simulink model "Smart_EV_Charging_Station_Project_Simulation"  (R2024b)
settings: Solver=ode23tb  StartTime=0.0  StopTime=4  RelTol=1e-12
undefined symbols (not defined in the file): Ion, Lithium
libraries: spsSeriesRLCBranchLib x34, spsPWMGeneratorDCDCLib x12, spsIdealSwitchLib x12, slpidlib x11, spsGroundLib x10, spsMosfetLib x10, spsIGBTDiodeLib x8, spsDiodeLib x7, spsVoltageMeasurementLib x7, spsBatteryLib x6, spsIGBTLib x6, spsThyristorLib x6
(part 1 of 3)
settings Model: Creator=HP  LastModifiedBy=mahad
settings SolverCC: AlgebraicLoopSolver=TrustRegion
settings DataIOCC: ReturnWorkspaceOutputs=off
settings DebuggingCC: UnconnectedInputMsg=warning  UnconnectedOutputMsg=warning  UnconnectedLineMsg=warning  ArithmeticOperatorsInVariantConditions=warning
settings ModelReferenceCC: EnableRefExpFcnMdlSchedulingChecks=on
settings SFSimCC: SimUseLocalCustomCode=off  CustomCodeUndefinedFunction=UseInterfaceOnly
settings RTWCC: RTWUseLocalCustomCode=off  GPUComputeCapability=3.5
settings CodeAppCC: StateflowObjectComments=on
settings SimscapeCC: SimscapeNormalizeSystem=off

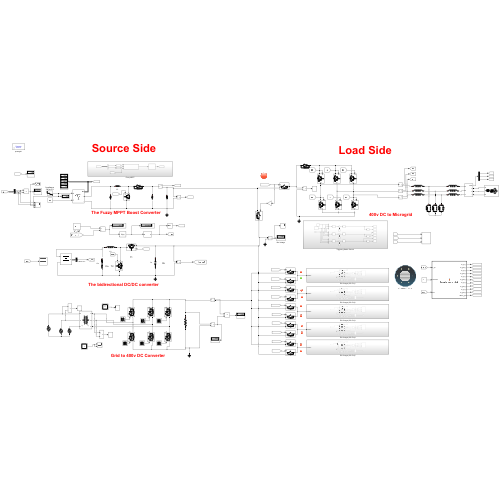
[thumbnail: Simulink's stored preview of the top-level diagram]
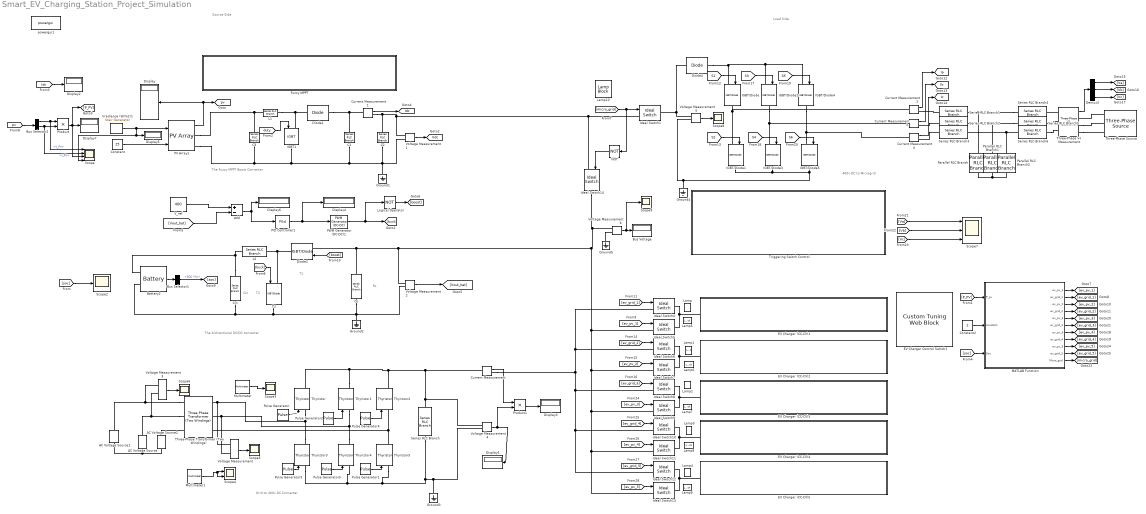
== system Smart_EV_Charging_Station_Project_Simulation ==
  note: The bidirectional DC/DC converter
  note: The Fuzzy MPPT Boost Converter
  note: Grid to 400v DC Converter
  note: 400v DC to Microgrid
  note: Source Side
  note: Load Side
  note: T1
  note: T2
  note: Cin
  note: RL
  AC Voltage Source : spsACVoltageSourceLib/AC Voltage Source  Amplitude=120*1.414  Phase=-120  Frequency=60  SampleTime=0  Measurements=Voltage  BusType=swing  Pref=10e3  Qref=0  Qmin=-inf  Qmax=+inf
  AC Voltage Source1 : spsACVoltageSourceLib/AC Voltage Source  Amplitude=120*1.414  Phase=0  Frequency=60  SampleTime=0  Measurements=Voltage  BusType=swing  Pref=10e3  Qref=0  Qmin=-inf  Qmax=+inf
  AC Voltage Source2 : spsACVoltageSourceLib/AC Voltage Source  Amplitude=120*1.414  Phase=-240  Frequency=60  SampleTime=0  Measurements=Voltage  BusType=swing  Pref=10e3  Qref=0  Qmin=-inf  Qmax=+inf
  Add : Sum  Inputs=+-
  Battery2 : spsBatteryLib/Battery  BatType=Lithium-Ion  NomV=400  NomQ=1400  SOC=50  Batt_Tr=0.01  PresetModel=on  MaxQ=1400  MinV=300  FullV=465.5949  Dis_rate=608.6957  R=0.0028571  Normal_OP=1266.087  expZone="[432.1543      68.78261]"
      settings: LibrarySourceBlock=electricdrivelib/Extra Sources/Battery
  Bus Selector1 : BusSelector  OutputSignals=SOC (%)
  Bus Selector2 : BusSelector  OutputSignals=V_PV,I_PV
  Bus Voltage : Display
  C1 : spsSeriesRLCBranchLib/Series RLC Branch  LConnTagsString=__new0  RConnTagsString=__new0  BranchType=C  Resistance=1.0  Inductance=1.0  SetiL0=off  InitialCurrent=0  Capacitance=0.04  Setx0=off  InitialVoltage=0  Measurements=None
  C2 : spsSeriesRLCBranchLib/Series RLC Branch  LConnTagsString=__new0  RConnTagsString=__new0  BranchType=R  Resistance=0.28  Inductance=1.0  SetiL0=off  InitialCurrent=0  Capacitance=100e-6  Setx0=off  InitialVoltage=0  Measurements=Branch voltage
  C3 : spsSeriesRLCBranchLib/Series RLC Branch  LConnTagsString=__new0  RConnTagsString=__new0  BranchType=C  Resistance=1.0  Inductance=1.0  SetiL0=off  InitialCurrent=0  Capacitance=0.00018  Setx0=off  InitialVoltage=0  Measurements=None
  Cin : spsSeriesRLCBranchLib/Series RLC Branch  LConnTagsString=__new0  RConnTagsString=__new0  BranchType=RC  Resistance=0.0000005  Inductance=3e-3  SetiL0=off  InitialCurrent=0  Capacitance=0.015  Setx0=off  InitialVoltage=0  Measurements=None
  Co : spsSeriesRLCBranchLib/Series RLC Branch  LConnTagsString=__new0  RConnTagsString=__new0  BranchType=C  Resistance=1  Inductance=3e-3  SetiL0=off  InitialCurrent=0  Capacitance=0.01  Setx0=off  InitialVoltage=0  Measurements=None
  Constant : Constant  Value=25
  Constant2 : Constant
  Current Measurement{,1..4} (5 alike) : spsCurrentMeasurementLib/Current Measurement  PhasorSimulation=off  OutputType=Complex  PSBequivalent=0
  Demux3 : Demux  Outputs=3
  Diode1 : spsDiodeLib/Diode  Ron=0.001  Lon=0  Vf=0.8  IC=0  UseSnubber=0  Rs=500  Cs=250e-9  Measurements=off
  Diode2 : spsIGBTDiodeLib/IGBT//Diode  Ron=1e-3  Rs=1e5  Cs=inf  Measurements=off
  Diode4 : spsDiodeLib/Diode  Ron=0.001  Lon=0  Vf=0.8  IC=0  UseSnubber=0  Rs=500  Cs=250e-9  Measurements=off
  Display{,1..7} (8 alike) : Display
  EV Charger (CC-CV)1 : Subsystem
  EV Charger (CC-CV)2 : Subsystem
  EV Charger (CC-CV)3 : Subsystem
  EV Charger (CC-CV)4 : Subsystem
  EV Charger (CC-CV)5 : Subsystem
  EV Charger Control Switch1 : CustomTuningWebBlock  LabelPosition=Bottom  ShowInitialText=on  Configuration="{\"components\":[{\"name\":\"RotarySwitchComponent\",\"settings\":{\"arcAngle\":300,\"arcAngleOffset\":120,\"handle\":{\"size\":[150,150],\"src\":\"data:image\\/svg+xml;base64,PHN2ZyBpZD0iTGF5ZXJfMSIgZGF0YS1uYW1lPSJMYXllciAxIiB4bWxucz0iaHR0cDovL3d3dy53My5vcmcvMjAwMC9zdmciIHhtbG5zOnhsaW5rPSJodHRwOi8vd3d3LnczLm9yZy8xOTk5L3hsaW5rIiB2aWV3Qm94PSIwIDAgMTIxIDEyMSI+PGRlZnM+PHN0eWxlPi5jbHMtMXtmaWxsOnVybCgjbGluZWFyLWdyYWRpZW50KTt9LmNscy0yLC5jbHMtM3tmaWxsOiNkMWQxZDE7fS5jbHMtM3tzdHJva2U6I2I3YjdiNztzdHJva2UtbWl0ZXJsaW1pdDoxMDtzdHJva2Utd2lkdGg6MC4yNXB4O30uY2xzLTR7ZmlsbDojZjMwMDAwO30uY2xzLTV7ZmlsbDojZjIxNzY3O308L3N0eWxlPjxsaW5lYXJHcmFkaWVudCBpZD0ibGluZWFyLWdyYWRpZW50IiB4MT0iNjAuNSIgeTE9IjEyMC41IiB4Mj0iNjAuNSIgeTI9IjAuNSIgZ3JhZGllbnRVbml0cz0idXNlclNwYWNlT25Vc2UiPjxzdG9wIG9mZnNldD0iMCIgc3RvcC1jb2xvcj0iI2QxZDFkMSIvPjxzdG9wIG9mZnNldD0iMC4xIiBzdG9wLWNvbG9yPSIjY2VjZWNlIi8+PHN0b3Agb2Zmc2V0PSIwLjE5IiBzdG9wLWNvbG9yPSIjYzNjM2MzIi8+PHN0b3Agb2Zmc2V0PSIwLjI4IiBzdG9wLWNvbG9yPSIjYjFiMWIxIi8+PHN0b3Agb2Zmc2V0PSIwLjM2IiBzdG9wLWNvbG9yPSIjOTg5ODk4Ii8+PHN0b3Agb2Zmc2V0PSIwLjQ0IiBzdG9wLWNvbG9yPSIjNzg3ODc4Ii8+PHN0b3Agb2Zmc2V0PSIwLjQ2IiBzdG9wLWNvbG9yPSIjNmI2YjZiIi8+PHN0b3Agb2Zmc2V0PSIwLjU0IiBzdG9wLWNvbG9yPSIjNmI2YjZiIi8+PHN0b3Agb2Zmc2V0PSIwLjU2IiBzdG9wLWNvbG9yPSIjNzY3Njc2Ii8+PHN0b3Agb2Zmc2V0PSIwLjY0IiBzdG9wLWNvbG9yPSIjOTc5Nzk3Ii8+PHN0b3Agb2Zmc2V0PSIwLjcyIiBzdG9wLWNvbG9yPSIjYjBiMGIwIi8+PHN0b3Agb2Zmc2V0PSIwLjgxIiBzdG9wLWNvbG9yPSIjYzNjM2MzIi8+PHN0b3Agb2Zmc2V0PSIwLjkiIHN0b3AtY29sb3I9IiNjZGNkY2QiLz48c3RvcCBvZmZzZXQ9IjEiIHN0b3AtY29sb3I9IiNkMWQxZDEiLz48L2xpbmVhckdyYWRpZW50PjwvZGVmcz48Y2lyY2xlIGNsYXNzPSJjbHMtMSIgY3g9IjYwLjUiIGN5PSI2MC41IiByPSI2MCIvPjxwYXRoIGNsYXNzPSJjbHMtMiIgZD0iTTYwLjUsMUE1OS41LDU5LjUsMCwxLDEsMSw2MC41LDU5LjU3LDU5LjU3LDAsMCwxLDYwLjUsMW0wLTFBNjAuNSw2MC41LDAsMSwwLDEyMSw2MC41LDYwLjUsNjAuNSwwLDAsMCw2MC41LDBaIi8+PHJlY3QgY2xhc3M9ImNscy0zIiB4PSIwLjUiIHk9IjUxLjUiIHdpZHRoPSIxMjAiIGhlaWdodD0iMTgiIHJ4PSIzLjA0Ii8+PHJlY3QgY2xhc3M9ImNscy00IiB4PSI1Ljc1IiB5PSI1OC43NSIgd2lkdGg9IjE2IiBoZWlnaHQ9IjMiLz48cGF0aCBjbGFzcz0iY2xzLTUiIGQ9Ik0yMS4yNSw1OS4yNXYyaC0xNXYtMmgxNW0xLTFoLTE3djRoMTd2LTRaIi8+PC9zdmc+\"},\"handleOffset\":[0,0],\"handleOrientation\":180,\"handlePosition\":[0,0,1,1],\"handleSize\":{\"height\":0.5,\"width\":0.5},\"labelRadius\":0.36,\"position\":[0,0,1,1],\"states\":[{\"Label\":{\"color\":[0,0,0,1],\"icon\":{\"size\":[0,0],\"src\":[],\"srcOrientation\":\"Right\"},\"iconOffset\":0,\"iconPlacement\":\"left\",\"opacity\":1,\"position\":[0.7345552884615385,0.6796274038461538],\"show\":true,\"text\":{\"content\":\"0\",\"font\":\"Helvetica\"}},\"Value\":0},{\"Label\":{\"color\":[0,0,0,1],\"icon\":{\"size\":[0,0],\"src\":[],\"srcOrientation\":\"Right\"},\"iconOffset\":0,\"iconPlacement\":\"left\",\"opacity\":1,\"position\":[0.35757211538461536,0.7603966346153846],\"show\":true,\"text\":{\"content\":\"1\",\"font\":\"Helvetica\"}},\"Value\":1},{\"Label\":{\"color\":[0,0,0,1],\"icon\":{\"size\":[0,0],\"src\":[],\"srcOrientation\":\"Right\"},\"iconOffset\":0,\"iconPlacement\":\"left\",\"opacity\":1,\"position\":[0.09603365384615385,0.46033653846153844],\"show\":true,\"text\":{\"content\":\"2\",\"font\":\"Helvetica\"}},\"Value\":2},{\"Label\":{\"color\":[0,0,0,1],\"icon\":{\"size\":[0,0],\"src\":[],\"srcOrientation\":\"Right\"},\"iconOffset\":0,\"iconPlacement\":\"left\",\"opacity\":1,\"position\":[0.36532451923076925,0.1180889423076923],\"show\":true,\"text\":{\"content\":\"3\",\"font\":\"Helvetica\"}},\"Value\":3},{\"Label\":{\"color\":[0,0,0,1],\"icon\":{\"size\":[0,0],\"src\":[],\"srcOrientation\":\"Right\"},\"iconOffset\":0,\"iconPlacement\":\"left\",\"opacity\":1,\"position\":[0.7191706730769231,0.19501201923076922],\"show\":true,\"text\":{\"content\":\"4\",\"font\":\"Helvetica\"}},\"Value\":4},{\"Label\":{\"color\":[0,0,0,1],\"icon\":{\"size\":[0,0],\"src\":[],\"srcOrientation\":\"Right\"},\"iconOffset\":0,\"iconPlacement\":\"left\",\"opacity\":1,\"position\":[0.7191706730769231,0.19501201923076922],\"show\":true,\"text\":{\"content\":\"5\",\"font\":\"Helvetica\"}},\"Value\":5}],\"tickRadius\":0.32}},{\"name\":\"BackgroundImageComponent\",\"settings\":{\"image\":{\"size\":[155,150],\"src\":\"data:image\\/svg+xml;base64,PD94bWwgdmVyc2lvbj0iMS4wIiBlbmNvZGluZz0idXRmLTgiPz4NCjwhLS0gR2VuZXJhdG9yOiBBZG9iZSBJbGx1c3RyYXRvciAyNS4wLjAsIFNWRyBFeHBvcnQgUGx1Zy1JbiAuIFNWRyBWZXJzaW9uOiA2LjAwIEJ1aWxkIDApICAtLT4NCjxzdmcgdmVyc2lvbj0iMS4xIg0KCSBpZD0iTGF5ZXJfMl8xXyIgeG1sbnM6Y2M9Imh0dHA6Ly9jcmVhdGl2ZWNvbW1vbnMub3JnL25zIyIgeG1sbnM6ZGM9Imh0dHA6Ly9wdXJsLm9yZy9kYy9lbGVtZW50cy8xLjEvIiB4bWxuczppbmtzY2FwZT0iaHR0cDovL3d3dy5pbmtzY2FwZS5vcmcv ...(+4184 chars)\",\"srcOrientation\":\"Right\"},\"position\":[0,0,1,1],\"scaleMode\":\"0\"}},{\"name\":\"ForegroundImageComponent\",\"settings\":{\"image\":{\"size\":[0,0],\"src\":\"default\",\"srcOrientation\":[]},\"isForeground\":1,\"position\":[0,0,1,1],\"scaleMode\":\"0\"}}],\"settings\":{\"BindingType\":\"param\",\"backgroundColor\":[0,0,255,\"1\"],\"backgroundOffset\":1,\"fixedAspectRatio\":\"on\",\"image\":{\"size\":[150,150],\"src\":\"data:image\\/svg+xml;base64,PD94bWwgdmVyc2lvbj0iMS4wIiBlbmNvZGluZz0iVVRGLTgiIHN0YW5kYWxvbmU9Im5vIj8+CjwhLS0gR2VuZXJhdG9yOiBBZG9iZSBJbGx1c3RyYXRvciAxOS4yLjEsIFNWRyBFeHBvcnQgUGx1Zy1JbiAuIFNWRyBWZXJzaW9uOiA2LjAwIEJ1aWxkIDApICAtLT4KCjxzdmcKICAgeG1sbnM6ZGM9Imh0dHA6Ly9wdXJsLm9yZy9kYy9lbGVtZW50cy8xLjEvIgogICB4bWxuczpjYz0iaHR0cDovL2NyZWF0aXZlY29tbW9ucy5vcmcvbnMjIgogICB4bWxuczpyZGY9Imh0dHA6Ly93d3cudzMub3JnLzE5OTkvMDIvMjItcmRmLXN5bnRh ...(+9660 chars)\"},\"showBackgroundColor\":false,\"variant\":\"rotarySwitch\",\"version\":\"R2023a\"},\"type\":\"RotarySwitch\"}"
  Fuzzy MPPT : Subsystem
  Ground{1..5} (5 alike) : spsGroundLib/Ground  LConnTagsString=a
  IGBT/Diode{,1..5} (6 alike) : spsIGBTDiodeLib/IGBT//Diode  Ron=1e-3  Rs=1e5  Cs=inf  Measurements=off
  IGBT1 : spsIGBTLib/IGBT  Ron=0.001  Lon=0  Vf=0  Tf=0  Tt=0  IC=0  Rs=1e5  Cs=inf  Measurements=off
  Ideal Switch{1,4..14} (12 alike) : spsIdealSwitchLib/Ideal Switch  Ron=0.001  Lon=0  IC=0  Rs=1e5  Cs=inf  Measurements=off
  Irradiance (W/m2)1 : spsStairGeneratorLib/Stair Generator  t=[0, 1, 2,3]  e=[1,0.8, 0.7, 0.6]*1000  Ts=0.0001
  L1 : spsSeriesRLCBranchLib/Series RLC Branch  LConnTagsString=__new0  RConnTagsString=__new0  BranchType=L  Resistance=0.005  Inductance=1.8e-05  SetiL0=off  InitialCurrent=0  Capacitance=1e-6  Setx0=off  InitialVoltage=0  Measurements=None
  L2 : spsSeriesRLCBranchLib/Series RLC Branch  LConnTagsString=__new0  RConnTagsString=__new0  BranchType=L  Resistance=.25  Inductance=4e-4  SetiL0=off  InitialCurrent=0  Capacitance=1e-6  Setx0=off  InitialVoltage=0  Measurements=None
  Lamp{,1..10} (11 alike) : LampBlock  LabelPosition=Hide
  Logical Operator : Logic  Operator=NOT  AllPortsSameDT=off  OutDataTypeStr=boolean
  MATLAB Function : MATLAB Function  TreatAsAtomicUnit=on
  Multimeter : spsMultimeterLib/Multimeter  L=11  sel=[2 3]  yselected={}  Gain=[1 1]  OutputType=Complex  PlotAtSimulationStop=off  PhasorSimulation=off
  Multimeter1 : spsMultimeterLib/Multimeter  L=11  sel=4  yselected={}  Gain=1  OutputType=Complex  PlotAtSimulationStop=off  PhasorSimulation=off
  NOT : Logic  Operator=NOT  IconShape=distinctive  AllPortsSameDT=off  OutDataTypeStr=boolean
  PID Controller1 : slpidlib/PID Controller  Controller=PI  Form=Parallel  TimeDomain=Continuous-time  UseExternalTs=off  SampleTime=-1  IntegratorMethod=Forward Euler  FilterMethod=Forward Euler  ControllerParametersSource=internal  P=0.00001  I=0.005  UseKiTs=off  D=0  UseExternalDerivativeSource=off  N=100  UseFilter=on  TunerSelectOption=Transfer Function Based (PID Tuner App)  InitialConditionSource=internal  InitialConditionForIntegrator=0  InitialConditionForFilter=0  DifferentiatorICPrevScaledInput=0  ExternalReset=none  TrackingMode=off  Kt=1  LimitOutput=off  SatLimitsSource=internal  UpperSaturationLimit=inf  LowerSaturationLimit=-inf  LinearizeAsGain=on  AntiWindupMode=none  Kb=1  LimitIntegrator=off  UpperIntegratorSaturationLimit=inf  LowerIntegratorSaturationLimit=-inf  POutMin=[]  POutMax=[]  IOutMin=[]  IOutMax=[]  DOutMin=[]  DOutMax=[]  NOutMin=[]  NOutMax=[]  SumOutMin=[]  SumOutMax=[]  SaturationOutMin=[]  SaturationOutMax=[]  PParamMin=[]  PParamMax=[]  IParamMin=[]  IParamMax=[]  DParamMin=[]  DParamMax=[]  NParamMin=[]  NParamMax=[]  KbParamMin=[]  KbParamMax=[]  KtParamMin=[]  KtParamMax=[]  KbOutMin=[]  KbOutMax=[]  KtOutMin=[]  KtOutMax=[]  IntegratorOutMin=[]  IntegratorOutMax=[]  FilterOutMin=[]  FilterOutMax=[]  SumI1OutMin=[]  SumI1OutMax=[]  SumI2OutMin=[]  SumI2OutMax=[]  SumI3OutMin=[]  SumI3OutMax=[]  SumI4OutMin=[]  SumI4OutMax=[]  SumDOutMin=[]  SumDOutMax=[]  DifferentiatorOutMin=[]  DifferentiatorOutMax=[]  FilterDiffOutCoefMin=[]  FilterDiffOutCoefMax=[]  ReciprocalOutMin=[]  ReciprocalOutMax=[]  SumDenOutMin=[]  SumDenOutMax=[]  SumNumOutMin=[]  SumNumOutMax=[]  DivideOutMin=[]  DivideOutMax=[]  UdiffTsProdOutMin=[]  UdiffTsProdOutMax=[]  NTsProdOutMin=[]  NTsProdOutMax=[]  UintegralTsProdOutMin=[]  UintegralTsProdOutMax=[]  UngainTsProdOutMin=[]  UngainTsProdOutMax=[]  ClampingZeroOutDataTypeStr=Inherit: Inherit via back propagation  ClampingZeroOutMin=[]  ClampingZeroOutMax=[]  FilterDenConstantOutDataTypeStr=Inherit: Inherit via back propagation  FilterDenConstantOutMin=[]  FilterDenConstantOutMax=[]  PCopyOutDataTypeStr=Inherit: Inherit via back propagation  PCopyOutMin=[]  PCopyOutMax=[]  NCopyOutDataTypeStr=Inherit: Inherit via back propagation  NCopyOutMin=[]  NCopyOutMax=[]  IntegratorContinuousStateAttributes=''  IntegratorStateMustResolveToSignalObject=off  IntegratorRTWStateStorageClass=Auto  FilterContinuousStateAttributes=''  FilterStateMustResolveToSignalObject=off  FilterRTWStateStorageClass=Auto  ParallelPVariant=InternalParameters  IdealPVariant=Disabled  IVariant=InternalParameters  DVariant=Disabled  IntegratorVariant=Continuous  SatVariant=Disabled  AWVariant=Passthrough  PCopyVariant=Disabled  TRVariant=Disabled  FdbkBlocksVariant=Forward  IdealPFdbkVariant=Disabled  SatFdbkVariant=Disabled  DerivativeFilterVariant=Disabled  NVariant=Disabled  NCopyVariant=Disabled_SignalSpec  FilterICVariant=Disabled  IntegratorICVariant=InternalICs  ExternalResetVariant=Disabled  TRSumVariant=Passthrough  SumFdbkVariant=Disabled  SumVariant=Sum_PI  TsampFilterVariant=InternalTs  TsampNgainVariant=Passthrough  TsampIntegralVariant=Disabled_SignalSpec  ExternalSaturationOutDataTypeStr=Inherit: Same as second input  DerivativeSourceVariant=Disabled  PreIntVariant=InternalPreInt
  PV Array1 : spsPVArrayLib/PV Array  Npar=200  Nser=8  PlotType=array @ 25 deg.C & specified irradiances  S_vec="[ 1000  800  600 400 200 ]"  Temp_C_vec="[ 45 25  ]"  ModuleName=Canadian Solar Inc. CS3U-375MS-AG  PlotWhenSelected=off  Pm=375.314  Ncell=72  Voc=47.6  Isc=9.93  Vm=39.8  Im=9.43  beta_Voc_pc=-0.293  alpha_Isc_pc=0.035005  beta_Voc=-0.13947  alpha_Isc=0.003476  IL=9.9881  I0=2.473e-11  nI=0.96345  Rsh=294.0017  Rs=0.24088  RobustModel=off  RobustCellTemperature=313.3991  BAL=off  Tc=1e-6  Tfilter=1e-5
  PWM Generator (DC-DC)1 : spsPWMGeneratorDCDCLib/PWM Generator (DC-DC)  Fsw=10000  Ts=0
  Parallel RLC Branch : spsParallelRLCBranchLib/Parallel RLC Branch  LConnTagsString=a  RConnTagsString=__new0  BranchType=RC  Resistance=5.34  Inductance=1e-3  SetiL0=off  InitialCurrent=0  Capacitance=9.94e-6  Setx0=off  InitialVoltage=0  Measurements=None
  Parallel RLC Branch1 : spsParallelRLCBranchLib/Parallel RLC Branch  LConnTagsString=a  RConnTagsString=__new0  BranchType=RC  Resistance=5.34  Inductance=1e-3  SetiL0=off  InitialCurrent=0  Capacitance=9.94e-6  Setx0=off  InitialVoltage=0  Measurements=None
  Parallel RLC Branch2 : spsParallelRLCBranchLib/Parallel RLC Branch  LConnTagsString=a  RConnTagsString=__new0  BranchType=RC  Resistance=5.34  Inductance=1e-3  SetiL0=off  InitialCurrent=0  Capacitance=9.94e-6  Setx0=off  InitialVoltage=0  Measurements=None
  Product : Product
  Product1 : Product
  Pulse Generator : DiscretePulseGenerator  PulseType=Time based  Period=0.016  PulseWidth=33.33  PhaseDelay=60*0.016/360
  Pulse Generator1 : DiscretePulseGenerator  PulseType=Time based  Period=0.016  PulseWidth=33.33  PhaseDelay=120*0.016/360
  Pulse Generator2 : DiscretePulseGenerator  PulseType=Time based  Period=0.016  PulseWidth=33.33  PhaseDelay=180*0.016/360
  Pulse Generator3 : DiscretePulseGenerator  PulseType=Time based  Period=0.016  PulseWidth=33.33  PhaseDelay=240*0.016/360
  Pulse Generator4 : DiscretePulseGenerator  PulseType=Time based  Period=0.016  PulseWidth=33.33  PhaseDelay=300*0.016/360
  Pulse Generator5 : DiscretePulseGenerator  PulseType=Time based  Period=0.016  PulseWidth=33.33  PhaseDelay=360*0.016/360
  Scope : Scope  NumInputPorts=4
  Scope{2..3,5..6,8..9} (6 alike) : Scope
  Scope4 : Scope  NumInputPorts=2
  Scope7 : Scope  NumInputPorts=3
  Series RLC Branch : spsSeriesRLCBranchLib/Series RLC Branch  LConnTagsString=__new0  RConnTagsString=__new0  BranchType=R  Resistance=10  Inductance=1e-3  SetiL0=off  InitialCurrent=0  Capacitance=1e-6  Setx0=off  InitialVoltage=0  Measurements=Branch voltage and current
  Series RLC Branch{1,4..6} (4 alike) : spsSeriesRLCBranchLib/Series RLC Branch  LConnTagsString=__new0  RConnTagsString=__new0  BranchType=L  Resistance=1e-3  Inductance=5.1e-3  SetiL0=off  InitialCurrent=0  Capacitance=1e-6  Setx0=off  InitialVoltage=0  Measurements=None
  Series RLC Branch2 : spsSeriesRLCBranchLib/Series RLC Branch  LConnTagsString=__new0  RConnTagsString=__new0  BranchType=L  Resistance=1e-3  Inductance=5.1e-6  SetiL0=off  InitialCurrent=0  Capacitance=1e-6  Setx0=off  InitialVoltage=0  Measurements=None
  Series RLC Branch3 : spsSeriesRLCBranchLib/Series RLC Branch  LConnTagsString=__new0  RConnTagsString=__new0  BranchType=L  Resistance=1e-3  Inductance=5.1e-6  SetiL0=off  InitialCurrent=0  Capacitance=1e-6  Setx0=off  InitialVoltage=0  Measurements=None
  T2 : spsIGBTDiodeLib/IGBT//Diode  Ron=1e-3  Rs=1e5  Cs=inf  Measurements=off
  Three-Phase Transformer (Two Windings) : spsThreePhaseTransformerTwoWindingsLib/Three-Phase Transformer (Two Windings)  Winding1Connection=Yg  Winding2Connection=Yg  CoreType=Three single-phase transformers  SetSaturation=off  Hysteresis=off  DataFile='hysteresis'  SetInitialFlux=off  Measurements=None  UNITS=pu  NominalPower=[ 1000e3 , 60 ]  Winding1=[ 296 , 0.002 , 0.08 ]  Winding2=[ 208 , 0.002 , 0.08 ]  Rm=500  Lm=500  L0=0.5  Saturation=[ 0,0 ; 0.0024,1.2 ; 1.0,1.52 ]  InitialFluxes=[ 0.8 , -0.8 , 0.7 ]  BreakLoop=off  DiscreteSolver=Trapezoidal iterative  DataType=off  TransfoNumber=1
  Three-Phase V-I Measurement : spsThreePhaseVIMeasurementLib/Three-Phase V-I Measurement  VoltageMeasurement=phase-to-phase  SetLabelV=off  LabelV=Vabc  Vpu=off  VpuLL=off  CurrentMeasurement=no  SetLabelI=off  LabelI=Iabc  Ipu=off  Pbase=100e6  Vbase=500e3  OutputType=Complex  PhasorSimulation=off  PSBequivalent=0
  Three-Phase Source : spsThreePhaseSourceLib/Three-Phase Source  InternalConnection=Y  VoltagePhases=off  Voltage=208  PhaseAngle=0  Voltage_phases=[25e3 25e3 25e3]/sqrt(3)  PhaseAngles_phases=[0 -120 +120]  Frequency=60  NonIdealSource=on  SpecifyImpedance=off  Resistance=0.001e-3  Inductance=0.001e-9  ShortCircuitLevel=100e6  BaseVoltage=208  XRratio=7  BusType=PQ  Pref=600000  Qref=0  Prefabc=[10e3, 10e3, 10e3]  Qrefabc=[0, 0, 0]  Qmin=-inf  Qmax=inf
  Thyristor{,1..5} (6 alike) : spsThyristorLib/Thyristor  Ron=0.001  Lon=0  Vf=0.8  IC=0  Rs=500  Cs=250e-9  Measurements=on
  Triggering Switch Control : Subsystem
  V_ref : Constant  Value=400
  Voltage Measurement{,1..6} (7 alike) : spsVoltageMeasurementLib/Voltage Measurement  PhasorSimulation=off  OutputType=Complex  PSBequivalent=0
  powergui1 : spspowerguiLib/powergui  Priority=1  SimulationMode=Discrete  SampleTime=1e-6  frequency=60  Iterations=50  frequencyindice=0  Pbase=100e6  ErrMax=1e-4  UnitsV=kV  UnitsW=MW  buscounter=0  FunctionMessages=off  echomessages=off  EnableUseOfTLC=off  CurrentSourceSwitches=off  DisableSnubberDevices=off  DisableRonSwitches=off  DisableVfSwitches=off  DisplayEquations=off  AutomaticDiscreteSolvers=off  SolverType=Tustin/Backward Euler (TBE)  Interpol=off  ExternalGateDelay=off  methode=off  Ts=100  x0status=blocks  SPID=on  SwTol=0  HookPort=off  NonlinearTolerance=1e-4  nMaxIteration=100  ContinueOnMaxIteration=off  RestoreLinks=warning  ResistiveCurrentMeasurement=off  Frange=[0:2:500]  Ylog=off  Xlog=on  ShowGrid=off  save=off  variable=ZData  structure=0  ZoomFFT=off  StartTime=0.0  cycles=1  DisplayStyle=1  fundamental=60  FreqAxis=off  MaxFrequency=1000  frequencyindicesteady=1  RmsSteady=1  display=off
  tag scope: Ia=global, Ib=global, Ic=global, Idc=global, Vdc=global, pv=global
  wires:
  Voltage Measurement1/1 -> [Vdc]
  [Idc] -> Display2/1
  Irradiance (W/m2)1/1 -> Scope/4, Display5/1, PV Array1/1
  Constant/1 -> PV Array1/2
  [duty] -> IGBT1/1
  Current Measurement1/1 -> [Idc]
  PV Array1/1 -> [pv], Display/1
  Pulse Generator5/1 -> Thyristor4/1
  Pulse Generator2/1 -> Thyristor1/1
  Pulse Generator/1 -> Thyristor/1
  Multimeter/1 -> Scope3/1
  Pulse Generator1/1 -> Thyristor5/1
  Voltage Measurement3/1 -> Scope6/1
  Voltage Measurement/1 -> Scope5/1
  Pulse Generator3/1 -> Thyristor3/1
  Pulse Generator4/1 -> Thyristor2/1
  Voltage Measurement4/1 -> Product1/2, Display1/1
  Multimeter1/1 -> Scope4/2, Scope4/1
  [S2] -> IGBT/Diode1/1
  Voltage Measurement5/1 -> Scope8/1
  Demux3/3 -> [Vc]
  Current Measurement3/1 -> [Ib]
  [S4] -> IGBT/Diode3/1
  [S5] -> IGBT/Diode4/1
  [Va] -> Scope7/1
  Current Measurement4/1 -> [Ic]
  [S1] -> IGBT/Diode/1
  Demux3/1 -> [Va]
  Three-Phase V-I Measurement/1 -> Demux3/1
  Current Measurement2/1 -> [Ia]
  [S3] -> IGBT/Diode2/1
  [S6] -> IGBT/Diode5/1
  Demux3/2 -> [Vb]
  [Vc] -> Scope7/3
  [micro_grid] -> NOT/1, Ideal Switch1/1
  [Vb] -> Scope7/2
  [buck] -> T2/1
  Battery2/1 -> Bus Selector1/1
  [boost] -> Diode2/1
  Bus Selector1/1 -> [soc]  "<SOC (%)>"
  Voltage Measurement2/1 -> [Vout_bat]
  [soc] -> Scope2/1
  Voltage Measurement6/1 -> Scope9/1, Bus Voltage/1
  NOT/1 -> Ideal Switch14/1
  Bus Selector2/2 -> Product/2, Scope/2  "<I_PV>"
  [pv] -> Bus Selector2/1
  Product/1 -> Scope/3, [P_PV], Display7/1
  Bus Selector2/1 -> Scope/1, Product/1  "<V_PV>"
  Logical Operator/1 -> [boost]
  PID Controller1/1 -> Display4/1, PWM Generator (DC-DC)1/1
  [Vout_bat] -> Add/2
  Add/1 -> PID Controller1/1, Display6/1
  V_ref/1 -> Add/1
  PWM Generator (DC-DC)1/1 -> Logical Operator/1, [buck]
  MATLAB Function/10(ev_grid_5) -> [ev_grid_5]
  MATLAB Function/5(ev_pv_3) -> [ev_pv_3]
  Constant2/1 -> MATLAB Function/2(constant)
  [ev_grid_1] -> Ideal Switch4/1
  [ev_pv_3] -> Ideal Switch9/1
  [ev_pv_2] -> Ideal Switch7/1
  [ev_pv_1] -> Ideal Switch5/1
  MATLAB Function/2(ev_grid_1) -> [ev_grid_1]
  [ev_grid_5] -> Ideal Switch12/1
  MATLAB Function/11(Micro_grid) -> [micro_grid]
  [ev_grid_4] -> Ideal Switch10/1
  [ev_pv_4] -> Ideal Switch11/1
  [ev_grid_2] -> Ideal Switch6/1
  [ev_grid_3] -> Ideal Switch8/1
  MATLAB Function/8(ev_grid_4) -> [ev_grid_4]
  MATLAB Function/4(ev_grid_2) -> [ev_grid_2]
  MATLAB Function/7(ev_pv_4) -> [ev_pv_4]
  [P_PV] -> MATLAB Function/1(P_pv)
  MATLAB Function/1(ev_pv_1) -> [ev_pv_1]
  MATLAB Function/6(ev_grid_3) -> [ev_grid_3]
  MATLAB Function/3(ev_pv_2) -> [ev_pv_2]
  [soc] -> MATLAB Function/3(Soc)
  [ev_pv_5] -> Ideal Switch13/1
  MATLAB Function/9(ev_pv_5) -> [ev_pv_5]
  Current Measurement/1 -> Product1/1
  Product1/1 -> Display3/1
  connections:
  IGBT1/RConn1 -- C3/RConn1 -- PV Array1/RConn2 -- C2/RConn1 -- Ground1/LConn1 -- Voltage Measurement1/LConn2 -- C1/RConn1
  C3/LConn1 -- L1/LConn1 -- PV Array1/RConn1
  Current Measurement1/LConn1 -- C1/LConn1 -- Diode1/RConn1
  Diode1/LConn1 -- IGBT1/LConn1 -- L1/RConn1
  Thyristor2/LConn1 -- Thyristor5/RConn1 -- Three-Phase Transformer (Two Windings)/LConn3
  Thyristor4/LConn1 -- Thyristor3/LConn1 -- Ground3/LConn1 -- Voltage Measurement4/LConn2 -- Series RLC Branch/RConn1 -- Thyristor5/LConn1
  Thyristor4/RConn1 -- Thyristor1/LConn1 -- Voltage Measurement/LConn2 -- Three-Phase Transformer (Two Windings)/LConn2
  Thyristor3/RConn1 -- Thyristor/LConn1 -- Voltage Measurement/LConn1 -- Three-Phase Transformer (Two Windings)/LConn1
  Three-Phase Transformer (Two Windings)/RConn2 -- AC Voltage Source/RConn1 -- Voltage Measurement3/LConn2
  AC Voltage Source1/LConn1 -- AC Voltage Source/LConn1 -- AC Voltage Source2/LConn1
  Three-Phase Transformer (Two Windings)/RConn1 -- AC Voltage Source1/RConn1 -- Voltage Measurement3/LConn1
  AC Voltage Source2/RConn1 -- Three-Phase Transformer (Two Windings)/RConn3
  Current Measurement2/LConn1 -- IGBT/Diode/RConn1 -- IGBT/Diode1/LConn1
  Parallel RLC Branch2/RConn1 -- Parallel RLC Branch/RConn1 -- Parallel RLC Branch1/RConn1
  Series RLC Branch3/RConn1 -- Series RLC Branch6/LConn1 -- Parallel RLC Branch2/LConn1
  IGBT/Diode3/RConn1 -- Ground4/LConn1 -- Voltage Measurement5/LConn2 -- IGBT/Diode5/RConn1 -- IGBT/Diode1/RConn1
  Current Measurement3/LConn1 -- IGBT/Diode2/RConn1 -- IGBT/Diode3/LConn1
  IGBT/Diode2/LConn1 -- Diode4/RConn1 -- IGBT/Diode/LConn1 -- IGBT/Diode4/LConn1
  Series RLC Branch4/LConn1 -- Series RLC Branch1/RConn1 -- Parallel RLC Branch/LConn1
  IGBT/Diode5/LConn1 -- IGBT/Diode4/RConn1 -- Current Measurement4/LConn1
  Series RLC Branch5/LConn1 -- Series RLC Branch2/RConn1 -- Parallel RLC Branch1/LConn1
  Three-Phase V-I Measurement/RConn3 -- Three-Phase Source/RConn3
  Three-Phase Source/RConn1 -- Three-Phase V-I Measurement/RConn1
  Series RLC Branch3/LConn1 -- Current Measurement4/RConn1
  Series RLC Branch6/RConn1 -- Three-Phase V-I Measurement/LConn3
  Series RLC Branch2/LConn1 -- Current Measurement3/RConn1
  Series RLC Branch1/LConn1 -- Current Measurement2/RConn1
  Three-Phase V-I Measurement/RConn2 -- Three-Phase Source/RConn2
  Series RLC Branch5/RConn1 -- Three-Phase V-I Measurement/LConn2
  Three-Phase V-I Measurement/LConn1 -- Series RLC Branch4/RConn1
  Voltage Measurement5/LConn1 -- Diode4/LConn1 -- Ideal Switch1/RConn1
  T2/RConn1 -- Cin/RConn1 -- Battery2/LConn2 -- Voltage Measurement2/LConn2 -- Ground2/LConn1 -- Co/RConn1
  L2/RConn1 -- Diode2/RConn1 -- T2/LConn1
  Cin/LConn1 -- Battery2/LConn1 -- L2/LConn1
  Ground5/LConn1 -- Voltage Measurement6/LConn2
  Ideal Switch5/LConn1 -- Ideal Switch14/RConn1 -- Voltage Measurement6/LConn1 -- Diode2/LConn1 -- Co/LConn1 -- Voltage Measurement2/LConn1 -- Ideal Switch13/LConn1 -- Ideal Switch11/LConn1 -- Ideal Switch9/LConn1 -- Ideal Switch7/LConn1
  Thyristor1/RConn1 -- Thyristor/RConn1 -- Current Measurement/LConn1 -- Voltage Measurement4/LConn1 -- Series RLC Branch/LConn1 -- Thyristor2/RConn1
  Ideal Switch7/RConn1 -- Ideal Switch6/RConn1 -- EV Charger (CC-CV)2/LConn1
  Ideal Switch9/RConn1 -- Ideal Switch8/RConn1 -- EV Charger (CC-CV)3/LConn1
  Ideal Switch5/RConn1 -- Ideal Switch4/RConn1 -- EV Charger (CC-CV)1/LConn1
  Ideal Switch12/RConn1 -- Ideal Switch13/RConn1 -- EV Charger (CC-CV)5/LConn1
  Ideal Switch10/RConn1 -- Ideal Switch11/RConn1 -- EV Charger (CC-CV)4/LConn1
  Ideal Switch10/LConn1 -- Ideal Switch12/LConn1 -- Current Measurement/RConn1 -- Ideal Switch4/LConn1 -- Ideal Switch6/LConn1 -- Ideal Switch8/LConn1
  Current Measurement1/RConn1 -- Voltage Measurement1/LConn1 -- Ideal Switch14/LConn1 -- Ideal Switch1/LConn1 -- C2/LConn1
